simulink model "Simulation_Fahrmodell_v3"  (R2023b)
settings: Solver=ode14x  StartTime=0.0  StopTime=600  FixedStep=0.005  RelTol=1e-3
values from neighbouring files (symbols this model uses):
  bat = bat.computePack()    [DoE_main.m]    (also in DoE_main_sensitivity.m)
  cp = cp.computeP4Map(val_P4, 0, val_P4_DM, 0, 0)    [DoE_main.m]    (also in DoE_main_sensitivity.m = cp.computeP4Map(P4, E2, P4_DM, E3, E4))
  gb = gb.computeShiftMaps()    [DoE_main.m]    (also in DoE_main_sensitivity.m)
  P4 = cfgNum(cfg, 'P4', 0)    [DoE_main_sensitivity.m]    (also in PowertrainConfig.m = 0)
  P4_DM = cfgNum(cfg, 'P4_DM', 0)    [DoE_main_sensitivity.m]    (also in PowertrainConfig.m = 0)
  pt = pt.setupHybrid()    [DoE_main.m]    (also in DoE_main_sensitivity.m)
  veh = VehicleConfig()    [DoE_main.m]    (also in DoE_main_sensitivity.m)
undefined symbols (not defined in the file or in its folder): cp_Zelle_JpkgK, Ice_derfacLoadDecrease_MAP, Ice_derfacLoadIncrease_MAP, Ice_n_axis, Ice_relLoadMax_CUR_n, Ice_relLoadMax_CUR_val, Ice_rl_axis_norm, seconds, SKO_STREET_CHAL, SKO_WHEEL_TYP_CHAL, slip_pacejka, T_init_degC, Track, TT_sliced, use_turbo_model, v_Fzg_init_kmph
libraries: nesl_utility x15, fl_lib x9
(part 2 of 6)

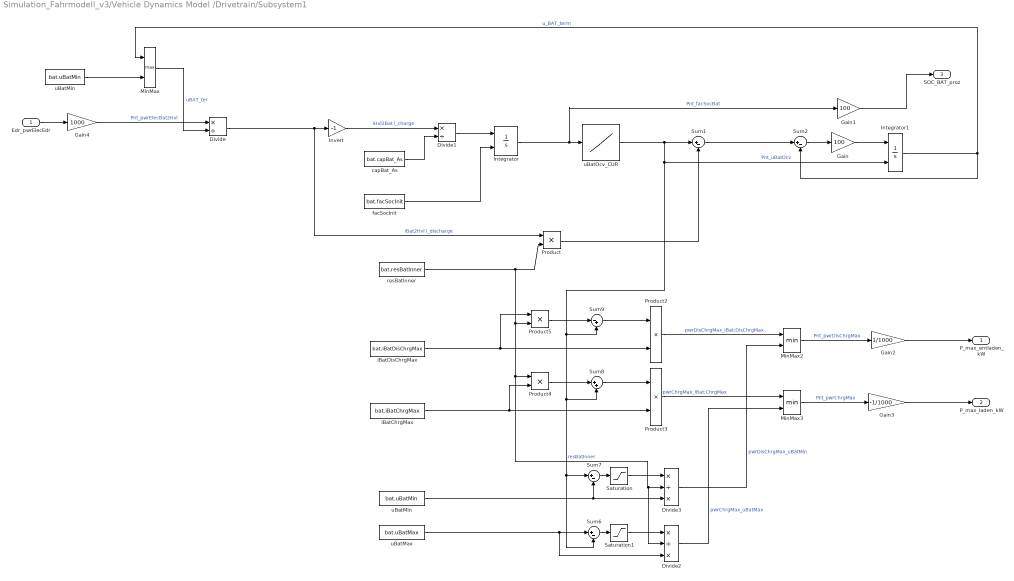
== system Simulation_Fahrmodell_v3/Vehicle Dynamics Model /Drivetrain/Subsystem1 ==
  Edr_pwrElecEdr : Inport
  Divide : Product  Inputs=*/
  Divide1 : Product  Inputs=*/
  Divide2 : Product  Inputs=*/*
  Divide3 : Product  Inputs=*/*
  Gain : Gain  Gain=100
  Gain1 : Gain  Gain=100
  Gain2 : Gain  Gain=1/1000
  Gain3 : Gain  Gain=-1/1000
  Gain4 : Gain  Gain=1000
  Integrator : Integrator  InitialConditionSource=external  InitialCondition=0.8  LimitOutput=on  UpperSaturationLimit=1  LowerSaturationLimit=0
  Integrator1 : Integrator  InitialConditionSource=external  InitialCondition=0.8
  Invert : Gain  Gain=-1
  MinMax : MinMax  Function=max  Inputs=2
  MinMax2 : MinMax  Inputs=2
  MinMax3 : MinMax  Inputs=2
  Product : Product  RndMeth=Zero
  Product{2..5} (4 alike) : Product
  Saturation : Saturate  UpperLimit=1000  LowerLimit=0
  Saturation1 : Saturate  UpperLimit=1000  LowerLimit=0
  Sum{1..2,6..7} (4 alike) : Sum  Inputs=|+-
  Sum8 : Sum  Inputs=|++
  Sum9 : Sum  Inputs=|-+
  capBat_As : Constant  Value=bat.capBat_As
  facSocInit : Constant  Value=bat.facSocInit
  iBatChrgMax : Constant  Value=bat.iBatChrgMax
  iBatDisChrgMax : Constant  Value=bat.iBatDisChrgMax
  resBatInner : Constant  Value=bat.resBatInner
  uBatMax : Constant  Value=bat.uBatMax
  uBatMin : Constant  Value=bat.uBatMin
  "uBatMin " : Constant  Value=bat.uBatMin
  uBatOcv_CUR : Lookup_n-D  NumberOfTableDimensions=1  BreakpointsForDimension1=bat.Soc_Axis  Table=bat.uBatOcv_Table  InternalRulePriority=Speed  RndMeth=Simplest
  P_max_entladen_kW : Outport  VectorParamsAs1DForOutWhenUnconnected=off
  P_max_laden_kW : Outport  Port=2  VectorParamsAs1DForOutWhenUnconnected=off
  SOC_BAT_proz : Outport  Port=3  VectorParamsAs1DForOutWhenUnconnected=off
  wires:
  Edr_pwrElecEdr/1 -> Gain4/1
  Gain4/1 -> Divide/1  "Pnt_pwrElecBat2Hvl"
  MinMax/1 -> Divide/2  "uBAT_ter"
  Divide/1 -> Product/1, Invert/1  "iBat2Hvl i_discharge"
  Invert/1 -> Divide1/1  "iHvl2Bat i_charge"
  capBat_As/1 -> Divide1/2
  facSocInit/1 -> Integrator/2
  Divide1/1 -> Integrator/1
  Integrator/1 -> Gain1/1, uBatOcv_CUR/1  "Pnt_facSocBat"
  uBatOcv_CUR/1 -> Sum9/2, Sum8/2, Sum7/1, Sum6/2, Integrator1/2, Sum1/1  "Pnt_uBatOcv"
  resBatInner/1 -> Product/2, Product5/2, Divide2/2, Divide3/2, Product4/1  "resBatInner"
  Product/1 -> Sum1/2
  iBatChrgMax/1 -> Product3/2, Product4/2
  iBatDisChrgMax/1 -> Product2/2, Product5/1
  Product5/1 -> Sum9/1
  Product4/1 -> Sum8/1
  Sum9/1 -> Product2/1
  Sum8/1 -> Product3/1
  Product2/1 -> MinMax2/1  "pwrDisChrgMax_iBat;DisChrgMax"
  Product3/1 -> MinMax3/1  "pwrChrgMax_iBat;ChrgMax"
  Saturation/1 -> Divide3/1
  Sum6/1 -> Saturation1/1
  uBatMax/1 -> Sum6/1, Divide2/3
  Saturation1/1 -> Divide2/1
  Sum7/1 -> Saturation/1
  "uBatMin "/1 -> Sum7/2, Divide3/3
  Divide3/1 -> MinMax2/2  "pwrDisChrgMax_uBatMin"
  Divide2/1 -> MinMax3/2  "pwrChrgMax_uBatMax"
  MinMax2/1 -> Gain2/1  "Pnt_pwrDisChrgMax"
  MinMax3/1 -> Gain3/1  "Pnt_pwrChrgMax"
  uBatMin/1 -> MinMax/2
  Integrator1/1 -> MinMax/1, Sum2/2  "u_BAT_term"
  Sum2/1 -> Gain/1
  Gain/1 -> Integrator1/1
  Sum1/1 -> Sum2/1
  Gain1/1 -> SOC_BAT_proz/1
  Gain2/1 -> P_max_entladen_kW/1
  Gain3/1 -> P_max_laden_kW/1

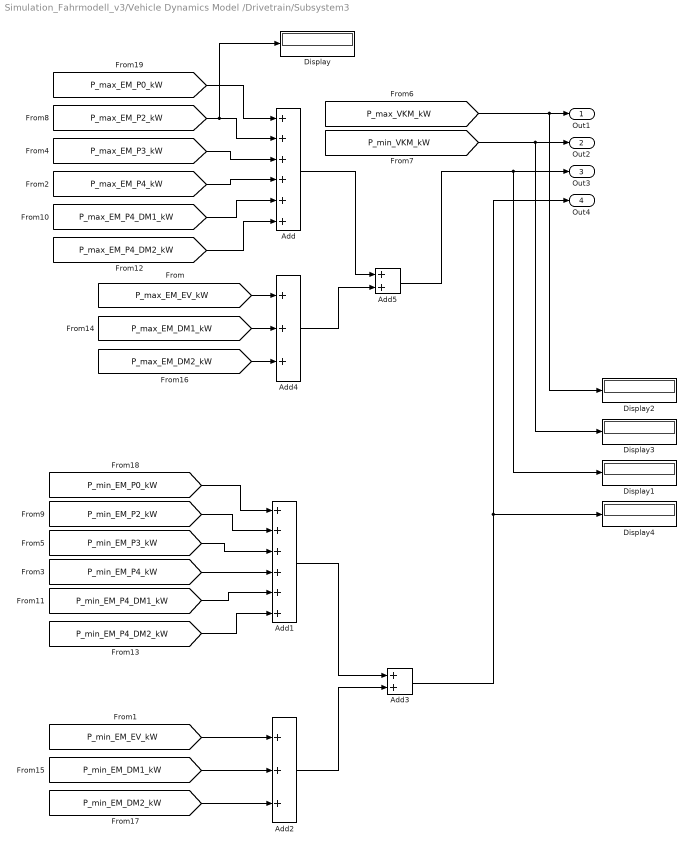
== system Simulation_Fahrmodell_v3/Vehicle Dynamics Model /Drivetrain/Subsystem3 ==
  Add : Sum  Inputs=++++++
  Add1 : Sum  Inputs=++++++
  Add2 : Sum  Inputs=+++
  Add3 : Sum
  Add4 : Sum  Inputs=+++
  Add5 : Sum
  Display{,1..4} (5 alike) : Display
  Out1 : Outport
  Out2 : Outport  Port=2
  Out3 : Outport  Port=3
  Out4 : Outport  Port=4
  wires:
  Add3/1 -> Out4/1, Display4/1
  Add1/1 -> Add3/1
  [P_min_EM_DM2_kW] -> Add2/3
  [P_min_EM_DM1_kW] -> Add2/2
  Add/1 -> Add5/1
  [P_max_EM_P4_DM1_kW] -> Add/5
  [P_max_EM_P3_kW] -> Add/3
  [P_max_EM_P0_kW] -> Add/1
  [P_max_EM_P2_kW] -> Add/2, Display/1
  [P_min_EM_EV_kW] -> Add2/1
  [P_min_EM_P4_DM2_kW] -> Add1/6
  [P_min_EM_P3_kW] -> Add1/3
  [P_max_EM_P4_kW] -> Add/4
  [P_max_EM_P4_DM2_kW] -> Add/6
  [P_min_EM_P0_kW] -> Add1/1
  Add2/1 -> Add3/2
  [P_min_VKM_kW] -> Out2/1, Display3/1
  [P_max_VKM_kW] -> Out1/1, Display2/1
  [P_min_EM_P4_DM1_kW] -> Add1/5
  [P_min_EM_P2_kW] -> Add1/2
  [P_min_EM_P4_kW] -> Add1/4
  [P_max_EM_DM1_kW] -> Add4/2
  [P_max_EM_EV_kW] -> Add4/1
  [P_max_EM_DM2_kW] -> Add4/3
  Add4/1 -> Add5/2
  Add5/1 -> Display1/1, Out3/1

== system Simulation_Fahrmodell_v3/Vehicle Dynamics Model /Drivetrain/Umrechung BAT -> EM 1 ==
  P_BAT_kW : Inport
  Add : Sum
  Constant6 : Constant  Value=0
  Gain4 : Gain  Gain=0.95
  Gain5 : Gain  Gain=0.95
  Gain6 : Gain  Gain=1/0.95
  Gain7 : Gain  Gain=1/0.95
  Max : MinMax  Function=max  Inputs=2
  Min4 : MinMax  Inputs=2
  P_EM_kW : Outport
  wires:
  Max/1 -> Gain4/1
  Constant6/1 -> Max/2, Min4/2
  P_BAT_kW/1 -> Max/1, Min4/1
  Gain5/1 -> Add/2
  Min4/1 -> Gain6/1
  Gain7/1 -> Add/1
  Add/1 -> P_EM_kW/1
  Gain6/1 -> Gain7/1
  Gain4/1 -> Gain5/1

== system Simulation_Fahrmodell_v3/Vehicle Dynamics Model /Drivetrain/Umrechung BAT -> EM 2 ==
  P_BAT_kW : Inport
  Add : Sum
  Constant6 : Constant  Value=0
  Gain4 : Gain  Gain=0.95
  Gain5 : Gain  Gain=0.95
  Gain6 : Gain  Gain=1/0.95
  Gain7 : Gain  Gain=1/0.95
  Max : MinMax  Function=max  Inputs=2
  Min4 : MinMax  Inputs=2
  P_EM_kW : Outport
  wires:
  Max/1 -> Gain4/1
  Constant6/1 -> Max/2, Min4/2
  P_BAT_kW/1 -> Max/1, Min4/1
  Gain5/1 -> Add/2
  Min4/1 -> Gain6/1
  Gain7/1 -> Add/1
  Add/1 -> P_EM_kW/1
  Gain6/1 -> Gain7/1
  Gain4/1 -> Gain5/1

== system Simulation_Fahrmodell_v3/Vehicle Dynamics Model /Drivetrain/Unterscheidung Regler und Gaspedal ==
  Regelfaktor : Inport
  Abs : Abs  SaturateOnIntegerOverflow=off
  Constant : Constant  Value=0
  Max : MinMax  Function=max  Inputs=2
  Gaspedalposition : Outport
  Regler : Outport  Port=2
  wires:
  Constant/1 -> Max/1
  Regelfaktor/1 -> Abs/1, Max/2
  Max/1 -> Gaspedalposition/1
  Abs/1 -> Regler/1

== system Simulation_Fahrmodell_v3/Vehicle Dynamics Model /Drivetrain/Wirkungsgrad Antriebsstrang Radebene -> Motorebene ==
  F_N IN : Inport
  Constant1 : Constant  Value=0.92
  Fahren : Product  Inputs=*/
  Reku : Product
  Switch1 : Switch  Criteria=u2 > Threshold  SaturateOnIntegerOverflow=off  InputSameDT=off
  F_N OUT : Outport
  wires:
  Constant1/1 -> Fahren/2, Reku/2
  F_N IN/1 -> Switch1/2, Fahren/1, Reku/1
  Reku/1 -> Switch1/3
  Switch1/1 -> F_N OUT/1
  Fahren/1 -> Switch1/1

== system Simulation_Fahrmodell_v3/Vehicle Dynamics Model /Drivetrain/v_mps -> v_kmph1 ==
  v_ist_mps IN : Inport
  Gain2 : Gain  Gain=3.6
  v_ist_kmph : Outport
  v_ist_mps OUT : Outport  Port=2
  wires:
  v_ist_mps IN/1 -> Gain2/1, v_ist_mps OUT/1
  Gain2/1 -> v_ist_kmph/1  "V_ist (km/h)"

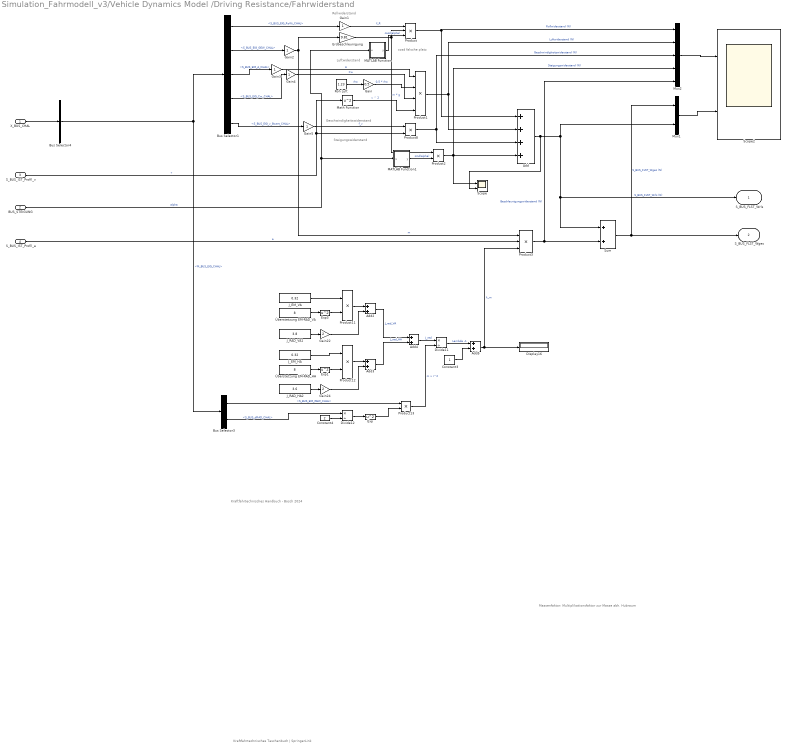
== system Simulation_Fahrmodell_v3/Vehicle Dynamics Model /Driving Resistance/Fahrwiderstand ==
  note: cosd falsche platz
  note: Kraftfahrtechnisches Taschenbuch | SpringerLink
  note: Kraftfahrtechnisches Handbuch - Bosch 2024
  note: Massenfaktor: Multiplikationsfaktor zur Masse abh. Hubraum
  note: Luftwiderstand
  note: Geschwindigkeitswiderstand
  note: Rollwiderstand
  note: Steigungswiderstand
  X_BUS_CHAL : Inport
  BUS_STEIGUNG : Inport  Port=2
  S_BUS_IST_Profil_v : Inport  Port=3
  S_BUS_IST_Profil_a : Inport  Port=4
  Add : Sum  Inputs=++++
  Add{2..5} (4 alike) : Sum
  Bus Selector1 : BusSelector  OutputSignals=S_BUS_EIG_RoWi_CHAL,S_BUS_EIG_GEW_CHAL,S_BUS_EIG_A_CHAL,S_BUS_EIG_Cw_CHAL,S_BUS_EIG_v_Bwert_CHAL
  Bus Selector3 : BusSelector  OutputSignals=S_BUS_EIG_GEW_CHAL,S_BUS_dRAD_CHAL
  Bus Selector4 : BusSelector  OutputSignals=M_BUS_EIG_CHAL
  Constant3 : Constant
  Constant4 : Constant  Value=2
  Display16 : Display
  Divide11 : Product  Inputs=*/
  Divide12 : Product  Inputs=*/
  Erdbeschleunigung : Gain  Gain=9.81
  Exp : Math  Operator=square
  Exp1 : Math  Operator=square
  Exp3 : Math  Operator=square
  Gain : Gain  Gain=0.5
  Gain{1..5} (5 alike) : Gain
  Gain22 : Gain  Gain=2
  Gain24 : Gain  Gain=2
  J_EM_HA : Constant  Value=0.32
  J_EM_VA : Constant  Value=0.32
  J_RAD_HA2 : Constant  Value=3.6
  J_RAD_VA1 : Constant  Value=3.8
  MATLAB Function : MATLAB Function  TreatAsAtomicUnit=on
  MATLAB Function1 : MATLAB Function  TreatAsAtomicUnit=on
  Math Function : Math  Operator=square
  Mux1 : Mux  Inputs=2
  Mux2 : Mux  Inputs=5
  Product : Product  Inputs=3
  Product1 : Product  Inputs=4
  Product{2,8,11..13} (5 alike) : Product
  Product3 : Product  Inputs=3
  Roh Luft : Constant  Value=1.23
  Scope : Scope  NumInputPorts=2
  Scope2 : Scope  NumInputPorts=2
  Sum : Sum
  Überstetzung EM-RAD_HA : Constant  Value=8
  Überstetzung EM-RAD_VA : Constant  Value=8
  S_BUS_FLST_Wrls : Outport
  S_BUS_FLST_Wges : Outport  Port=2
  wires:
  S_BUS_IST_Profil_a/1 -> Product3/2  "a"
  Bus Selector1/1 -> Gain1/1  "<S_BUS_EIG_RoWi_CHAL>"
  MATLAB Function/1(y) -> Product/3  "cosd(alpha)"
  Exp/1 -> Product13/2
  Math Function/1 -> Product1/4  "v ^ 2"
  MATLAB Function1/1(y) -> Product2/2  "sind(alpha)"
  BUS_STEIGUNG/1 -> MATLAB Function1/1(u), MATLAB Function/1(u)  "alpha"
  Bus Selector1/2 -> Gain2/1  "<S_BUS_EIG_GEW_CHAL>"
  Bus Selector1/3 -> Gain3/1  "<S_BUS_EIG_A_CHAL>"
  Product11/1 -> Add2/1
  Sum/1 -> S_BUS_FLST_Wges/1, Mux1/1  "S_BUS_FLST_Wges (N)"
  Erdbeschleunigung/1 -> Product2/1, Product/2  "m * g"
  Product13/1 -> Divide11/2  "m x r^2"
  Roh Luft/1 -> Gain/1  "rho"
  Product2/1 -> Add/4, Scope/1, Mux2/4  "Steigungswiderstand (N)"
  Product3/1 -> Sum/2, Mux2/5  "Beschleunigungswiderstand (N)"
  S_BUS_IST_Profil_v/1 -> Product8/2, Math Function/1  "v"
  Gain24/1 -> Add3/2
  Add/1 -> Scope/2, Mux1/2, Sum/1, S_BUS_FLST_Wrls/1  "S_BUS_FLST_Wrls (N)"
  Gain22/1 -> Add2/2
  J_EM_VA/1 -> Product11/1
  Mux2/1 -> Scope2/1
  Constant3/1 -> Add5/2
  Exp1/1 -> Product12/2
  Bus Selector1/5 -> Gain5/1  "<S_BUS_EIG_v_Bwert_CHAL>"
  Exp3/1 -> Product11/2
  Mux1/1 -> Scope2/2
  Bus Selector1/4 -> Gain4/1  "<S_BUS_EIG_Cw_CHAL>"
  Add4/1 -> Divide11/1  "J_red"
  Constant4/1 -> Divide12/2
  Product1/1 -> Mux2/2, Add/2  "Luftwiderstand (N)"
  Product/1 -> Add/1, Mux2/1  "Rollwiderstand (N)"
  Bus Selector3/2 -> Divide12/1  "<S_BUS_dRAD_CHAL>"
  Product12/1 -> Add3/1
  Gain/1 -> Product1/2  "0,5 * rho"
  Add2/1 -> Add4/1  "J_red_VA"
  Überstetzung EM-RAD_HA/1 -> Exp1/1
  J_RAD_VA1/1 -> Gain22/1
  Add5/1 -> Product3/3, Display16/1  "k_m"
  Add3/1 -> Add4/2  "J_rad_HA"
  J_EM_HA/1 -> Product12/1
  Divide12/1 -> Exp/1
  J_RAD_HA2/1 -> Gain24/1
  Überstetzung EM-RAD_VA/1 -> Exp3/1
  Product8/1 -> Add/3, Mux2/3  "Geschwindigkeitswiderstand (N)"
  Divide11/1 -> Add5/1  "Lambda -1"
  Bus Selector3/1 -> Product13/1  "<S_BUS_EIG_GEW_CHAL>"
  Bus Selector4/1 -> Bus Selector1/1, Bus Selector3/1  "<M_BUS_EIG_CHAL>"
  X_BUS_CHAL/1 -> Bus Selector4/1
  Gain1/1 -> Product/1  "f_R"
  Gain2/1 -> Product3/1, Erdbeschleunigung/1  "m"
  Gain3/1 -> Product1/1  "A"
  Gain4/1 -> Product1/3  "Cw"
  Gain5/1 -> Product8/1  "f_v"

== system Simulation_Fahrmodell_v3/Vehicle Dynamics Model /Driving Resistance/Subsystem ==
  X_BUS_CHAL : Inport
  BUS_STEIGUNG : Inport  Port=2
  M_m_Nm : Inport  Port=3
  Bus Selector2 : BusSelector  OutputSignals=M_BUS_EIG_CHAL.S_BUS_dRAD_CHAL
  Constant : Constant
  Delay1 : Delay  DelayLength=1
  Display{1..8} (8 alike) : Display
  Divide1 : Product  Inputs=*/
  Divide2 : Product  Inputs=*/
  Fahrwiderstand1 : Subsystem
  Integrator : Integrator
  Limit output 0..1 : Saturate  UpperLimit=1  LowerLimit=0
  Minus1 : Sum  Inputs=+-
  Minus2 : Sum  Inputs=+-
  Product{,1..3} (4 alike) : Product
  Scope2 : Scope  NumInputPorts=2
  Scope3 : Scope  NumInputPorts=2
  Test Konstante red. Massenträgheit : Constant  Value=65.92
  Tire Friction Model Pacejka Dry_tarmac : Lookup_n-D  NumberOfTableDimensions=1  BreakpointsForDimension1=slip_pacejka.Dry_tarmac.slip  Table=slip_pacejka.Dry_tarmac.y  UseLastTableValue=on  InternalRulePriority=Speed  RndMeth=Simplest
  "d -> r" : Gain  Gain=0.5
  g : Constant  Value=9.81
  m_kg : Constant  Value=2500
  wires:
  X_BUS_CHAL/1 -> Bus Selector2/1, Fahrwiderstand1/1(X_BUS_CHAL)
  M_m_Nm/1 -> Display2/1, Scope3/1, Minus2/1
  Fahrwiderstand1/1(v) -> Display8/1, Divide2/1  "v"
  Divide1/1 -> Integrator/1, Display1/1  "Winkelbeschleunigung Rad alpha_F"
  Divide2/1 -> Minus1/2
  Product3/1 -> Delay1/1  "Tire Force Disturbance"
  Minus1/1 -> Display4/1, Scope2/1, Limit output 0..1/1
  Test Konstante red. Massenträgheit/1 -> Divide1/2
  Tire Friction Model Pacejka Dry_tarmac/1 -> Display6/1, Product2/2  "Reibkoeffizient mu"
  "d -> r"/1 -> Display7/1, Product3/2, Product/2  "r"
  g/1 -> Product1/2
  Delay1/1 -> Scope3/2, Minus2/2, Display3/1
  m_kg/1 -> Product1/1
  Minus2/1 -> Divide1/1
  Limit output 0..1/1 -> Display5/1, Scope2/2, Tire Friction Model Pacejka Dry_tarmac/1  "Schlupf lambda"
  Bus Selector2/1 -> "d -> r"/1  "<S_BUS_dRAD_CHAL>"
  BUS_STEIGUNG/1 -> Fahrwiderstand1/2(BUS_STEIGUNG)
  Product2/1 -> Fahrwiderstand1/3(F_x_N), Product3/1  "F_x_N"
  Integrator/1 -> Product/1  "Winkelgeschwindigkeit Rad omega_F"
  Constant/1 -> Minus1/1
  Product1/1 -> Product2/1  "F_z_N"
  Product/1 -> Divide2/2  "omega_F * r"

== system Simulation_Fahrmodell_v3/Vehicle Properties/Fzg.-Eigenschaften/Eingabe i_GET und n_max_Upmin Andere Angaben ==
  Bus Creator : BusCreator  Inputs=8
  Bus Creator1 : BusCreator  Inputs=2
  Bus Creator2 : BusCreator  Inputs=8
  i_G1 : Constant  Value=i_G1
  i_G2 : Constant  Value=i_G2
  i_G3 : Constant  Value=i_G3
  i_G4 : Constant  Value=i_G4
  i_G5 : Constant  Value=i_G5
  i_G6 : Constant  Value=i_G6
  i_G7 : Constant  Value=i_G7
  i_G8 : Constant  Value=i_G8
  n_max_Upmin G1 : Constant  Value=n_max_Upmin_G1
  n_max_Upmin G2 : Constant  Value=n_max_Upmin_G2
  n_max_Upmin G3 : Constant  Value=n_max_Upmin_G3
  n_max_Upmin G4 : Constant  Value=n_max_Upmin_G4
  n_max_Upmin G5 : Constant  Value=n_max_Upmin_G5
  n_max_Upmin G6 : Constant  Value=n_max_Upmin_G6
  n_max_Upmin G7 HARTE GRENZE : Constant  Value=n_max_Upmin_G7
  n_max_Upmin G8 : Constant  Value=n_max_Upmin_G8
  BUS OUT : Outport
  wires:
  i_G1/1 -> Bus Creator/1  "G1"
  i_G2/1 -> Bus Creator/2  "G2"
  i_G3/1 -> Bus Creator/3  "G3"
  i_G4/1 -> Bus Creator/4  "G4"
  i_G5/1 -> Bus Creator/5  "G5"
  i_G6/1 -> Bus Creator/6  "G6"
  i_G7/1 -> Bus Creator/7  "G7"
  i_G8/1 -> Bus Creator/8  "G8"
  n_max_Upmin G1/1 -> Bus Creator2/1  "G1"
  n_max_Upmin G2/1 -> Bus Creator2/2  "G2"
  n_max_Upmin G6/1 -> Bus Creator2/6  "G6"
  n_max_Upmin G4/1 -> Bus Creator2/4  "G4"
  n_max_Upmin G3/1 -> Bus Creator2/3  "G3"
  n_max_Upmin G7 HARTE GRENZE/1 -> Bus Creator2/7  "G7"
  n_max_Upmin G5/1 -> Bus Creator2/5  "G5"
  n_max_Upmin G8/1 -> Bus Creator2/8  "G8"
  Bus Creator/1 -> Bus Creator1/1  "i_GET"
  Bus Creator2/1 -> Bus Creator1/2  "n_max_Upmin"
  Bus Creator1/1 -> BUS OUT/1

== system Simulation_Fahrmodell_v3/Vehicle Properties/Fzg.-Eigenschaften/Eingabe i_GET und n_max_Upmin Audi RS3 8YA PA ==
  Bus Creator : BusCreator  Inputs=8
  Bus Creator1 : BusCreator  Inputs=2
  Bus Creator2 : BusCreator  Inputs=8
  i_G1 : Constant  Value=i_G1
  i_G2 : Constant  Value=i_G2
  i_G3 : Constant  Value=i_G3
  i_G4 : Constant  Value=i_G4
  i_G5 : Constant  Value=i_G5
  i_G6 : Constant  Value=i_G6
  i_G7 : Constant  Value=i_G7
  i_G8 : Constant  Value=i_G8
  n_max_Upmin G1 : Constant  Value=n_max_Upmin_G1
  n_max_Upmin G2 : Constant  Value=n_max_Upmin_G2
  n_max_Upmin G3 : Constant  Value=n_max_Upmin_G3
  n_max_Upmin G4 : Constant  Value=n_max_Upmin_G4
  n_max_Upmin G5 : Constant  Value=n_max_Upmin_G5
  n_max_Upmin G6 : Constant  Value=n_max_Upmin_G6
  n_max_Upmin G7 HARTE GRENZE : Constant  Value=n_max_Upmin_G7
  n_max_Upmin G8 : Constant  Value=n_max_Upmin_G8
  BUS OUT : Outport
  wires:
  i_G1/1 -> Bus Creator/1  "G1"
  i_G2/1 -> Bus Creator/2  "G2"
  i_G3/1 -> Bus Creator/3  "G3"
  i_G4/1 -> Bus Creator/4  "G4"
  i_G5/1 -> Bus Creator/5  "G5"
  i_G6/1 -> Bus Creator/6  "G6"
  i_G7/1 -> Bus Creator/7  "G7"
  i_G8/1 -> Bus Creator/8  "G8"
  n_max_Upmin G1/1 -> Bus Creator2/1  "G1"
  n_max_Upmin G2/1 -> Bus Creator2/2  "G2"
  n_max_Upmin G6/1 -> Bus Creator2/6  "G6"
  n_max_Upmin G4/1 -> Bus Creator2/4  "G4"
  n_max_Upmin G3/1 -> Bus Creator2/3  "G3"
  n_max_Upmin G7 HARTE GRENZE/1 -> Bus Creator2/7  "G7"
  n_max_Upmin G5/1 -> Bus Creator2/5  "G5"
  n_max_Upmin G8/1 -> Bus Creator2/8  "G8"
  Bus Creator/1 -> Bus Creator1/1  "i_GET"
  Bus Creator2/1 -> Bus Creator1/2  "n_max_Upmin"
  Bus Creator1/1 -> BUS OUT/1

== system Simulation_Fahrmodell_v3/Vehicle Properties/Fzg.-Eigenschaften/Eingabe i_GET und n_max_Upmin Spreizung 7,0 ==
  Bus Creator : BusCreator  Inputs=8
  Bus Creator1 : BusCreator  Inputs=2
  Bus Creator2 : BusCreator  Inputs=8
  i_G1 : Constant  Value=i_G1
  i_G2 : Constant  Value=i_G2
  i_G3 : Constant  Value=i_G3
  i_G4 : Constant  Value=i_G4
  i_G5 : Constant  Value=i_G5
  i_G6 : Constant  Value=i_G6
  i_G7 : Constant  Value=i_G7
  i_G8 : Constant  Value=i_G8
  n_max_Upmin G1 : Constant  Value=n_max_Upmin_G1
  n_max_Upmin G2 : Constant  Value=n_max_Upmin_G2
  n_max_Upmin G3 : Constant  Value=n_max_Upmin_G3
  n_max_Upmin G4 : Constant  Value=n_max_Upmin_G4
  n_max_Upmin G5 : Constant  Value=n_max_Upmin_G5
  n_max_Upmin G6 : Constant  Value=n_max_Upmin_G6
  n_max_Upmin G7 HARTE GRENZE : Constant  Value=n_max_Upmin_G7
  n_max_Upmin G8 : Constant  Value=n_max_Upmin_G8
  BUS OUT : Outport
  wires:
  i_G1/1 -> Bus Creator/1  "G1"
  i_G2/1 -> Bus Creator/2  "G2"
  i_G3/1 -> Bus Creator/3  "G3"
  i_G4/1 -> Bus Creator/4  "G4"
  i_G5/1 -> Bus Creator/5  "G5"
  i_G6/1 -> Bus Creator/6  "G6"
  i_G7/1 -> Bus Creator/7  "G7"
  i_G8/1 -> Bus Creator/8  "G8"
  n_max_Upmin G1/1 -> Bus Creator2/1  "G1"
  n_max_Upmin G2/1 -> Bus Creator2/2  "G2"
  n_max_Upmin G6/1 -> Bus Creator2/6  "G6"
  n_max_Upmin G4/1 -> Bus Creator2/4  "G4"
  n_max_Upmin G3/1 -> Bus Creator2/3  "G3"
  n_max_Upmin G7 HARTE GRENZE/1 -> Bus Creator2/7  "G7"
  n_max_Upmin G5/1 -> Bus Creator2/5  "G5"
  n_max_Upmin G8/1 -> Bus Creator2/8  "G8"
  Bus Creator/1 -> Bus Creator1/1  "i_GET"
  Bus Creator2/1 -> Bus Creator1/2  "n_max_Upmin"
  Bus Creator1/1 -> BUS OUT/1

== system Simulation_Fahrmodell_v3/Vehicle Properties/Fzg.-Eigenschaften/Eingabe i_GET und n_max_Upmin Spreizung 7,8 ==
  Bus Creator : BusCreator  Inputs=8
  Bus Creator1 : BusCreator  Inputs=2
  Bus Creator2 : BusCreator  Inputs=8
  i_G1 : Constant  Value=i_G1
  i_G2 : Constant  Value=i_G2
  i_G3 : Constant  Value=i_G3
  i_G4 : Constant  Value=i_G4
  i_G5 : Constant  Value=i_G5
  i_G6 : Constant  Value=i_G6
  i_G7 : Constant  Value=i_G7
  i_G8 : Constant  Value=i_G8
  n_max_Upmin G1 : Constant  Value=n_max_Upmin_G1
  n_max_Upmin G2 : Constant  Value=n_max_Upmin_G2
  n_max_Upmin G3 : Constant  Value=n_max_Upmin_G3
  n_max_Upmin G4 : Constant  Value=n_max_Upmin_G4
  n_max_Upmin G5 : Constant  Value=n_max_Upmin_G5
  n_max_Upmin G6 : Constant  Value=n_max_Upmin_G6
  n_max_Upmin G7 HARTE GRENZE : Constant  Value=n_max_Upmin_G7
  n_max_Upmin G8 : Constant  Value=n_max_Upmin_G8
  BUS OUT : Outport
  wires:
  i_G1/1 -> Bus Creator/1  "G1"
  i_G2/1 -> Bus Creator/2  "G2"
  i_G3/1 -> Bus Creator/3  "G3"
  i_G4/1 -> Bus Creator/4  "G4"
  i_G5/1 -> Bus Creator/5  "G5"
  i_G6/1 -> Bus Creator/6  "G6"
  i_G7/1 -> Bus Creator/7  "G7"
  i_G8/1 -> Bus Creator/8  "G8"
  n_max_Upmin G1/1 -> Bus Creator2/1  "G1"
  n_max_Upmin G2/1 -> Bus Creator2/2  "G2"
  n_max_Upmin G6/1 -> Bus Creator2/6  "G6"
  n_max_Upmin G4/1 -> Bus Creator2/4  "G4"
  n_max_Upmin G3/1 -> Bus Creator2/3  "G3"
  n_max_Upmin G7 HARTE GRENZE/1 -> Bus Creator2/7  "G7"
  n_max_Upmin G5/1 -> Bus Creator2/5  "G5"
  n_max_Upmin G8/1 -> Bus Creator2/8  "G8"
  Bus Creator/1 -> Bus Creator1/1  "i_GET"
  Bus Creator2/1 -> Bus Creator1/2  "n_max_Upmin"
  Bus Creator1/1 -> BUS OUT/1

== system Simulation_Fahrmodell_v3/Environment/Nürburgring (M. Siesmann)/Vehicle Dynamics: Desired Speed (Kamm Circle)/Subsystem ==
  Clock2 : Clock
  Delay1 : Delay  DelayLength=1
  Minus1 : Sum  Inputs=+-
  delta_t_s : Outport
  wires:
  Delay1/1 -> Minus1/2
  Clock2/1 -> Delay1/1, Minus1/1
  Minus1/1 -> delta_t_s/1

== system Simulation_Fahrmodell_v3/Vehicle Dynamics Model /Drivetrain/Axle Load and Torque Distribution /Axle Torque Channel Router  ==
  Tq_Primary_axle : Inport
  Tq_Secondary_axle : Inport  Port=2
  Constant : Constant  Value=veh.HM_VA
  Constant1 : Constant  Value=0
  Constant3 : Constant  Value=pt.P4
  Constant4 : Constant  Value=pt.P4_DM
  OR1 : Logic  Operator=OR  IconShape=distinctive  AllPortsSameDT=off  OutDataTypeStr=boolean
  Switch{,1..4} (5 alike) : Switch  Criteria=u2 > Threshold  SaturateOnIntegerOverflow=off  InputSameDT=off
  Tq_FrontAxle : Outport
  Tq_RearAxle : Outport  Port=2
  wires:
  Tq_Primary_axle/1 -> Switch3/3, Switch1/3, Switch2/3, Switch/1
  Switch/1 -> Switch3/1
  Tq_Secondary_axle/1 -> Switch1/1, Switch/3
  Constant/1 -> Switch/2, Switch1/2
  Switch1/1 -> Switch2/1
  Switch2/1 -> Tq_RearAxle/1
  Switch4/1 -> Switch3/2, Switch2/2
  Switch3/1 -> Tq_FrontAxle/1
  Constant1/1 -> Switch4/1
  [P4_Deactivate] -> Switch4/2
  OR1/1 -> Switch4/3
  Constant3/1 -> OR1/1
  Constant4/1 -> OR1/2

== system Simulation_Fahrmodell_v3/Vehicle Dynamics Model /Drivetrain/Axle Load and Torque Distribution /Berechnung Max. Radlast VA//HA aufgrund Reifen//Fahrbahn ==
  F_Haftgrenze [N] : Inport
  Raddurchmesser [m] : Inport  Port=2
  axle_load_FrontAxle [%] : Inport  Port=3
  axle_load_RearAxle [%] : Inport  Port=4
  Gain : Gain  Gain=0.01
  Gain1 : Gain  Gain=0.01
  Product : Product
  Product1 : Product
  Radlast HA : Product
  Radlast VA : Product
  Scope : Scope  NumInputPorts=2
  Scope1 : Scope  NumInputPorts=2
  "d -> r" : Gain  Gain=0.5
  Max. Radlast VA [Nm] aufgrund Reifen/Fahrbahn : Outport
  Max. Radlast HA [Nm] aufgrund Reifen/Fahrbahn : Outport  Port=2
  wires:
  axle_load_FrontAxle [%]/1 -> Gain/1
  axle_load_RearAxle [%]/1 -> Gain1/1
  Radlast HA/1 -> Product1/1
  Radlast VA/1 -> Product/1
  F_Haftgrenze [N]/1 -> Scope1/1, Radlast VA/1, Radlast HA/1
  "d -> r"/1 -> Product1/2, Product/2
  Raddurchmesser [m]/1 -> "d -> r"/1
  Product/1 -> Scope/1, Max. Radlast VA [Nm] aufgrund Reifen/Fahrbahn/1
  Product1/1 -> Max. Radlast HA [Nm] aufgrund Reifen/Fahrbahn/1, Scope/2
  Gain/1 -> Radlast VA/2
  Gain1/1 -> Radlast HA/2

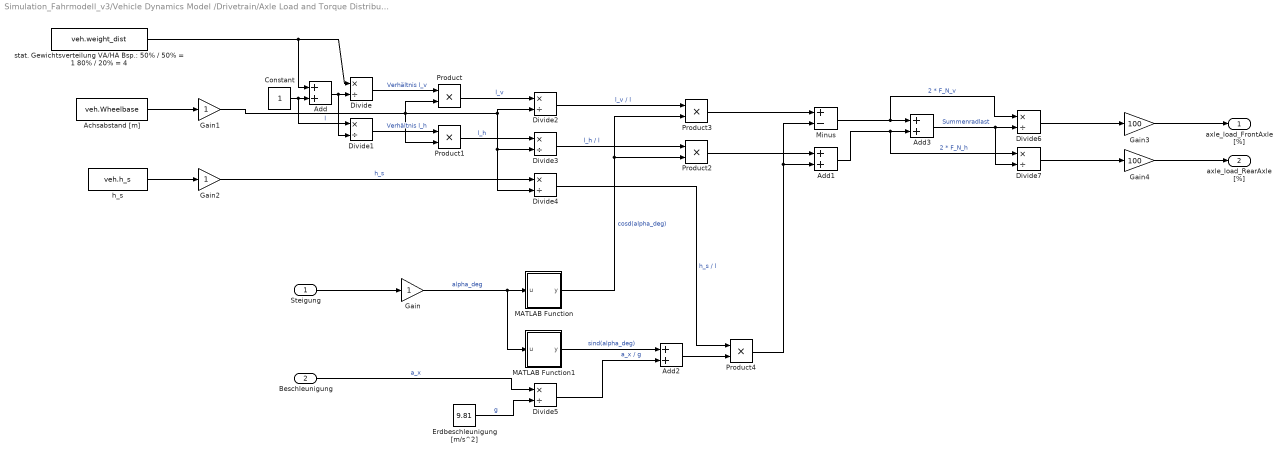
== system Simulation_Fahrmodell_v3/Vehicle Dynamics Model /Drivetrain/Axle Load and Torque Distribution /Berechnung Achslastverteilung abh. Fahrzeugeigenschaften (Haken Abs. 11) ==
  Steigung : Inport
  Beschleunigung : Inport  Port=2
  Achsabstand [m] : Constant  Value=veh.Wheelbase
  Add{,1..3} (4 alike) : Sum
  Constant : Constant
  Divide{,1..7} (8 alike) : Product  Inputs=*/
  Erdbeschleunigung [m/s^2] : Constant  Value=9.81
  Gain : Gain
  Gain1 : Gain
  Gain2 : Gain
  Gain3 : Gain  Gain=100
  Gain4 : Gain  Gain=100
  MATLAB Function : MATLAB Function  TreatAsAtomicUnit=on
  MATLAB Function1 : MATLAB Function  TreatAsAtomicUnit=on
  Minus : Sum  Inputs=+-
  Product{,1..4} (5 alike) : Product
  h_s : Constant  Value=veh.h_s
  stat. Gewichtsverteilung VA/HA Bsp.: 50% / 50% = 1 80% / 20% = 4 : Constant  Value=veh.weight_dist
  axle_load_FrontAxle [%] : Outport
  axle_load_RearAxle [%] : Outport  Port=2
  wires:
  Gain/1 -> MATLAB Function1/1(u), MATLAB Function/1(u)  "alpha_deg"
  Achsabstand [m]/1 -> Gain1/1
  Gain1/1 -> Divide4/2, Divide3/2, Divide2/2, Product1/2, Product/2  "l"
  Constant/1 -> Divide1/1, Add/2
  Add/1 -> Divide1/2, Divide/2
  stat. Gewichtsverteilung VA/HA Bsp.: 50% / 50% = 1 80% / 20% = 4/1 -> Divide/1, Add/1
  Divide/1 -> Product/1  "Verhältnis l_v"
  Divide1/1 -> Product1/1  "Verhältnis l_h"
  Product/1 -> Divide2/1  "l_v"
  Product1/1 -> Divide3/1  "l_h"
  MATLAB Function/1(y) -> Product3/2, Product2/2  "cosd(alpha_deg)"
  MATLAB Function1/1(y) -> Add2/1  "sind(alpha_deg)"
  Divide2/1 -> Product3/1  "l_v / l"
  Divide3/1 -> Product2/1  "l_h / l"
  h_s/1 -> Gain2/1
  Gain2/1 -> Divide4/1  "h_s"
  Divide4/1 -> Product4/1  "h_s / l"
  Beschleunigung/1 -> Divide5/1  "a_x"
  Erdbeschleunigung [m/s^2]/1 -> Divide5/2  "g"
  Divide5/1 -> Add2/2  "a_x / g"
  Product3/1 -> Minus/1
  Product2/1 -> Add1/1
  Add2/1 -> Product4/2
  Product4/1 -> Minus/2, Add1/2
  Minus/1 -> Divide6/1, Add3/1  "2 * F_N_v"
  Add1/1 -> Divide7/1, Add3/2  "2 * F_N_h"
  Divide6/1 -> Gain3/1
  Steigung/1 -> Gain/1
  Add3/1 -> Divide7/2, Divide6/2  "Summenradlast"
  Gain3/1 -> axle_load_FrontAxle [%]/1
  Divide7/1 -> Gain4/1
  Gain4/1 -> axle_load_RearAxle [%]/1

== system Simulation_Fahrmodell_v3/Vehicle Dynamics Model /Drivetrain/Axle Load and Torque Distribution /Drive Topology Axle Load Distributor  ==
  axle_load_FrontAxle [%] : Inport
  axle_load_RearAxle [%] : Inport  Port=2
  Tq_max_FrontAxle : Inport  Port=3
  Tq_max_RearAxle : Inport  Port=4
  Angetriebene Räder 1: Allrad 2: Hinterradantrieb 3: Vorderradantrieb : Constant  Commented=on  Value=3
  Constant : Constant  Value=0
  Constant1 : Constant  Value=0
  Constant2 : Constant  Value=pt.P4
  Constant3 : Constant  Value=veh.HM_VA
  Constant4 : Constant  Value=veh.AWD
  Constant5 : Constant  Value=pt.P4_DM
  Display : Display
  Display1 : Display
  Display2 : Display
  "Front Axle Load Calculator " : Subsystem
  MATLAB Function : MATLAB Function  TreatAsAtomicUnit=on
  Min2 : MinMax  Inputs=2
  Min3 : MinMax  Inputs=2
  Multiport Switch : MultiPortSwitch  SaturateOnIntegerOverflow=off  InputSameDT=off
  Multiport Switch1 : MultiPortSwitch  SaturateOnIntegerOverflow=off  InputSameDT=off
  OR1 : Logic  Operator=OR  IconShape=distinctive  AllPortsSameDT=off  OutDataTypeStr=boolean
  P4 AWD or AWD : Subsystem
  P4 AWD or AWD1 : Subsystem
  "Rear Axle Load Calculator " : Subsystem
  M_VA_Nm OUT : Outport
  M_HA_Nm OUT : Outport  Port=2
  wires:
  axle_load_FrontAxle [%]/1 -> "Rear Axle Load Calculator "/2(Achslast VA [%])
  Tq_max_RearAxle/1 -> "Rear Axle Load Calculator "/1(M_Nm), Min3/2, P4 AWD or AWD1/2(M_VA_Nm IN), Multiport Switch1/3
  "Rear Axle Load Calculator "/1(Radlast VA [Nm]) -> Min2/2
  Tq_max_FrontAxle/1 -> "Front Axle Load Calculator "/1(M_Nm), Multiport Switch/4, P4 AWD or AWD/1(M_VA_Nm IN), Min2/1
  axle_load_RearAxle [%]/1 -> "Front Axle Load Calculator "/2(Achslast HA [%])
  "Front Axle Load Calculator "/1(Radlast HA [Nm]) -> Min3/1
  Min2/1 -> Display/1, P4 AWD or AWD/2(In3)
  MATLAB Function/1(Driven_Wheels_Val) -> Multiport Switch1/1, Multiport Switch/1
  Multiport Switch/1 -> M_VA_Nm OUT/1
  Multiport Switch1/1 -> M_HA_Nm OUT/1
  Min3/1 -> P4 AWD or AWD1/3(In3), Display1/1
  Constant/1 -> Multiport Switch/3
  Constant1/1 -> Multiport Switch1/4
  Constant3/1 -> MATLAB Function/2(FWD)
  Constant4/1 -> MATLAB Function/1(AWD)
  Constant5/1 -> OR1/2
  Constant2/1 -> OR1/1
  OR1/1 -> P4 AWD or AWD1/1(In2), P4 AWD or AWD/3(In2), Display2/1, MATLAB Function/3(Check_P4)
  P4 AWD or AWD/1(Out1) -> Multiport Switch/2
  P4 AWD or AWD1/1(Out1) -> Multiport Switch1/2

== system Simulation_Fahrmodell_v3/Vehicle Dynamics Model /Drivetrain/Axle Load and Torque Distribution /Subsystem ==
  In1 : Inport
  In2 : Inport  Port=2
  "Tq_FrontAxle " : Inport  Port=3
  "Tq_RearAxle " : Inport  Port=4
  Gain{,1..3} (4 alike) : Gain  Gain=-1
  Max. Achslast HA [Nm] aufgrund Bauteilschutz : Constant  Value=8900
  Max. Achslast VA [Nm] aufgrund Bauteilschutz : Constant  Value=99999
  Min : MinMax  Inputs=3
  Min1 : MinMax  Inputs=3
  Min2 : MinMax  Function=max  Inputs=3
  Min3 : MinMax  Function=max  Inputs=3
  Tq_max_FrontAxle : Outport
  Tq_max_RearAxle : Outport  Port=2
  wires:
  Gain1/1 -> Min2/3
  Min/1 -> Min2/1
  In1/1 -> Min/2, Gain/1
  In2/1 -> Gain2/1, Min1/2
  Min1/1 -> Min3/1
  Max. Achslast HA [Nm] aufgrund Bauteilschutz/1 -> Gain3/1, Min1/3
  Gain3/1 -> Min3/3
  Max. Achslast VA [Nm] aufgrund Bauteilschutz/1 -> Gain1/1, Min/3
  Gain2/1 -> Min3/2
  Gain/1 -> Min2/2
  Min2/1 -> Tq_max_FrontAxle/1  "M_VA_Nm IN"
  "Tq_FrontAxle "/1 -> Min/1
  Min3/1 -> Tq_max_RearAxle/1  "M_HA_Nm IN"
  "Tq_RearAxle "/1 -> Min1/1

== system Simulation_Fahrmodell_v3/Vehicle Dynamics Model /Drivetrain/GETRIEBE auswahl VK, EV/Subsystem ==
  d_Rad_m : Inport
  Display4 : Display
  "d -> r" : Gain  Gain=0.5
  "m -> mm" : Gain  Gain=1000
  r_dyn_mm : Outport
  wires:
  d_Rad_m/1 -> "m -> mm"/1, Display4/1
  "d -> r"/1 -> r_dyn_mm/1
  "m -> mm"/1 -> "d -> r"/1

== system Simulation_Fahrmodell_v3/Vehicle Dynamics Model /Drivetrain/GETRIEBE auswahl VK, EV/Transmission Selector ==
  note: 1) Add Subsystem or Model blocks as valid variant choices.
      | 2) You cannot connect blocks at this level. At simulation, connectivity is automatically
      | determined, based on the active variant and port name matching.
  n_mot_Upmin : Inport
  i_AG : Inport  Port=2
  "Gaspedalposition [0, 1]" : Inport  Port=3
  " EV Single-Speed" : Subsystem  VariantControl=veh.EV == 1
  ICE Multi-Speed : Subsystem  VariantControl=veh.VM == 1 || veh.Hy ==1
  i_GES : Outport
  i_GES_delay : Outport  Port=2

== system Simulation_Fahrmodell_v3/Vehicle Dynamics Model /Drivetrain/GETRIEBE auswahl VK, EV/v_Fzg_kmph -> n_mot_Upmin ==
  i_GES : Inport
  r_dyn_mm : Inport  Port=2
  v_Fzg_kmph : Inport  Port=3
  Radschlupf : Inport  Port=4
  Constant : Constant  Value=2*pi*60/1000
  Divide : Product  Inputs=*/
  Product : Product
  Product1 : Product
  Product2 : Product
  "mm -> m" : Gain  Gain=0.001
  n_mot_Upmin : Outport
  wires:
  Product2/1 -> Product/1  "v_ist (km/h)"
  Radschlupf/1 -> Product2/1  "v_ist (km/h)"
  Divide/1 -> n_mot_Upmin/1
  Product1/1 -> Divide/2
  Constant/1 -> Product1/2
  Product/1 -> Divide/1
  i_GES/1 -> Product/2
  v_Fzg_kmph/1 -> Product2/2
  "mm -> m"/1 -> Product1/1
  r_dyn_mm/1 -> "mm -> m"/1

== system Simulation_Fahrmodell_v3/Vehicle Dynamics Model /Drivetrain/Operating Strategy 1.1/Axle Torque Split ==
  tq_wheel_des : Inport
  SOC : Inport  Port=2
  Add : Sum
  Constant1 : Constant  Value=pt.cfg_P4
  Constant2 : Constant  Value=veh.MainAxle_TorqueSplit_int
  Constant3 : Constant  Value=pt.cfg_P4_DM
  Constant4 : Constant  Value=gb.i_ges_P4
  Constant5 : Constant  Value=veh.EV
  Display : Display
  Display1 : Display
  Gain2 : Gain  Gain=0.01
  MATLAB Function1 : MATLAB Function  TreatAsAtomicUnit=on
  Min : MinMax  Inputs=2
  OR : Logic  Operator=OR  IconShape=distinctive  AllPortsSameDT=off  OutDataTypeStr=boolean
  Product : Product
  Product1 : Product
  Product4 : Product
  Saturation : Saturate  UpperLimit=10000  LowerLimit=0
  Subtract : Sum  Inputs=+-
  tq_wheel_Primary_axle_des : Outport
  tq_wheel_Secondary_axle_des : Outport  Port=2
  tag scope: P4_Deactivate=global
  wires:
  Product4/1 -> Min/2, Subtract/2  "tq_wheel_P4_max"
  Min/1 -> Display/1, tq_wheel_Secondary_axle_des/1  "tq_wheel_P4_des"
  Saturation/1 -> Add/2
  [tq_sh_P4_max] -> Product4/1
  Constant4/1 -> Product4/2
  Subtract/1 -> Saturation/1
  Add/1 -> tq_wheel_Primary_axle_des/1  "tq_wheel_ICEaxle_des"
  Product/1 -> Add/1  "tq_wheel_ICEaxle_des"
  Product1/1 -> Min/1, Subtract/1  "tq_wheel_P4axle_des"
  tq_wheel_des/1 -> Product1/2, Product/2  "tq_wheel_des"
  MATLAB Function1/2(Torque_ICE_Axle_percent) -> Product/1
  MATLAB Function1/3(Torque_P4_Axle_percent) -> Product1/1
  SOC/1 -> Gain2/1
  OR/1 -> MATLAB Function1/2(cfg_P4)
  Constant2/1 -> MATLAB Function1/4(MainAxle_TorqueSplit_int)
  Gain2/1 -> MATLAB Function1/1(SOC)
  Constant1/1 -> OR/1
  Constant3/1 -> OR/2
  Constant5/1 -> MATLAB Function1/3(EV)
  MATLAB Function1/1(P4_deactivate) -> [P4_Deactivate], Display1/1

== system Simulation_Fahrmodell_v3/Vehicle Dynamics Model /Drivetrain/Operating Strategy 1.1/EMs Priority (Ep) ==
  tq_wheel_Primary_axle_des : Inport
  i_ges : Inport  Port=2
  i_AG : Inport  Port=3
  SOC : Inport  Port=4
  Add1 : Sum  Inputs=+++
  Add2 : Sum  Inputs=+-
  MATLAB Function : MATLAB Function  TreatAsAtomicUnit=on  SystemSampleTime=0.01
  Min1 : MinMax  Inputs=2
  Product1 : Product
  Product2 : Product
  Product3 : Product
  SOC LIMIT : Subsystem  Commented=on
  Saturation : Saturate  UpperLimit=inf  LowerLimit=0
  tq_wheel_Elec_des_Ep : Outport
  tq_wheel_ICE_des_Ep : Outport  Port=2
  wires:
  tq_wheel_Primary_axle_des/1 -> Add2/1, Min1/2
  i_ges/1 -> Product2/1, Product1/1
  Add1/1 -> Min1/1, Add2/2
  [tq_sh_P2_max] -> Product2/2
  Product2/1 -> Add1/2  "tq_wheel_P2_max"
  Add2/1 -> Saturation/1
  Product3/1 -> Add1/3  "tq_wheel_P3_max"
  [tq_sh_P3_max] -> Product3/2
  Product1/1 -> Add1/1  "tq_wheel_P0_max"
  [tq_sh_P0_max] -> Product1/2
  i_AG/1 -> Product3/1
  Saturation/1 -> MATLAB Function/1(tq_ICE_in)  "tq_wheel_ICE_des_Ep"
  SOC/1 -> MATLAB Function/3(SOC)
  Min1/1 -> MATLAB Function/2(tq_Elec_in)  "tq_wheel_Elec_des_Ep"
  MATLAB Function/1(tq_ICE_out) -> tq_wheel_ICE_des_Ep/1
  MATLAB Function/2(tq_Elec_out) -> tq_wheel_Elec_des_Ep/1

== system Simulation_Fahrmodell_v3/Vehicle Dynamics Model /Drivetrain/Operating Strategy 1.1/ICE Priority (ICEp) ==
  tq_wheel_Primary_axle_des : Inport
  i_ges : Inport  Port=2
  Add : Sum  Inputs=+-
  Min : MinMax  Inputs=2
  Product : Product
  Saturation : Saturate  UpperLimit=inf  LowerLimit=0
  tq_wheel_Elec_des_ICEp : Outport
  tq_wheel_ICE_des_ICEp : Outport  Port=2
  wires:
  [tq_sh_ICE_max] -> Product/2
  tq_wheel_Primary_axle_des/1 -> Min/1, Add/1
  Min/1 -> tq_wheel_ICE_des_ICEp/1  "tq_wheel_ICE_des"
  Add/1 -> Saturation/1
  Saturation/1 -> tq_wheel_Elec_des_ICEp/1  "tq_wheel_Elec_des"
  Product/1 -> Min/2, Add/2  "tq_wheel_ICE_max"
  i_ges/1 -> Product/1

== system Simulation_Fahrmodell_v3/Vehicle Dynamics Model /Drivetrain/Operating Strategy 1.1/Priority Mode Output Combiner ==
  tq_wheel_Elec_des_ICEp : Inport
  tq_wheel_ICE_des_ICEp : Inport  Port=2
  tq_wheel_Elec_des_Ep : Inport  Port=3
  tq_wheel_ICE_des_Ep : Inport  Port=4
  Add : Sum
  Constant1 : Constant  Value=veh.VM
  Constant3 : Constant  Value=veh.Hybrid_ICE_priority
  Switch1 : Switch  Criteria=u2 > Threshold  SaturateOnIntegerOverflow=off  InputSameDT=off
  Switch2 : Switch  Criteria=u2 > Threshold  SaturateOnIntegerOverflow=off  InputSameDT=off
  Switch3 : Switch  Criteria=u2 > Threshold  SaturateOnIntegerOverflow=off  InputSameDT=off
  tq_wheel_ICE_des : Outport
  tq_wheel_Elec_des : Outport  Port=2
  wires:
  Add/1 -> Switch3/1
  Switch2/1 -> Switch3/3, Add/2
  Switch1/1 -> tq_wheel_Elec_des/1, Add/1
  Constant3/1 -> Switch1/2, Switch2/2
  tq_wheel_ICE_des_ICEp/1 -> Switch2/1
  tq_wheel_Elec_des_ICEp/1 -> Switch1/1
  tq_wheel_ICE_des_Ep/1 -> Switch2/3
  tq_wheel_Elec_des_Ep/1 -> Switch1/3
  Switch3/1 -> tq_wheel_ICE_des/1  "tq_wheel_ICE_des"
  Constant1/1 -> Switch3/2

== system Simulation_Fahrmodell_v3/Vehicle Dynamics Model /Drivetrain/Operating Strategy 1.1/Wheel-to-Shaft Converter and Demand Validators  ==
  i_ges : Inport
  i_AG : Inport  Port=2
  tq_wheel_ICE_des : Inport  Port=3
  tq_wheel_P0_des : Inport  Port=4
  tq_wheel_P2_des : Inport  Port=5
  tq_wheel_P3_des : Inport  Port=6
  tq_wheel_Primary_axle_des : Inport  Port=7
  tq_wheel_Secondary_axle_des : Inport  Port=8
  Bus Creator : BusCreator  Inputs=6
  Constant3 : Constant  Value=gb.i_ges_P4
  Constant4 : Constant  Value=gb.i_GET_EV
  Divide{,1..5} (6 alike) : Product  Inputs=*/
  EV Primary Axle Torque Path Selector : Subsystem
  Secondary Axle Torque Path Selector : Subsystem
  tq_sh_des : Outport
  wires:
  i_ges/1 -> Divide/2, Divide1/2, Divide3/2
  tq_wheel_ICE_des/1 -> Divide3/1
  tq_wheel_P3_des/1 -> Divide2/1
  tq_wheel_P0_des/1 -> Divide/1
  Constant3/1 -> Divide4/2
  i_AG/1 -> Divide2/2
  tq_wheel_P2_des/1 -> Divide1/1
  Divide1/1 -> Bus Creator/3  "tq_sh_P2_des"
  Divide3/1 -> Bus Creator/1  "tq_sh_ICE_des"
  Divide/1 -> Bus Creator/2  "tq_sh_P0_des"
  Divide2/1 -> Bus Creator/4  "tq_sh_P3_des"
  Divide4/1 -> Bus Creator/5  "tq_sh_P4_des"
  Divide5/1 -> Bus Creator/6  "tq_sh_EV_des"
  Bus Creator/1 -> tq_sh_des/1
  tq_wheel_Primary_axle_des/1 -> Secondary Axle Torque Path Selector/1(tq_wheel_Primary_axle_des), EV Primary Axle Torque Path Selector/1(tq_wheel_Primary_axle_des)
  Constant4/1 -> Divide5/2
  EV Primary Axle Torque Path Selector/1(tq_wheel_EV_des) -> Divide5/1
  tq_wheel_Secondary_axle_des/1 -> Secondary Axle Torque Path Selector/2(tq_wheel_Secondary_axle_des)
  Secondary Axle Torque Path Selector/1(tq_wheel_P4_des) -> Divide4/1

== system Simulation_Fahrmodell_v3/Vehicle Dynamics Model /Drivetrain/Primary and Secondary Axle Powertrain Selector/Primary Axle Powertrain Selector ==
  note: 1) Add Subsystem or Model blocks as valid variant choices.
      | 2) You cannot connect blocks at this level. At simulation, connectivity is automatically
      | determined, based on the active variant and port name matching.
  i_ges : Inport
  iAG : Inport  Port=2
  n_mot_Upmin : Inport  Port=3
  Regelfaktor : Inport  Port=4
  Torque_sh : Inport  Port=5
  Electric Drive : Subsystem  VariantControl=veh.EV == 1
  Hybrid Drive : Subsystem  VariantControl=veh.Hy == 1 || veh.VM == 1
  Tq_Primary_axle : Outport

== system Simulation_Fahrmodell_v3/Vehicle Dynamics Model /Drivetrain/Primary and Secondary Axle Powertrain Selector/Secondary Axle Powertrain Selector ==
  Regelfaktor1 : Inport
  n_mot_Upmin : Inport  Port=2
  iAG : Inport  Port=3
  i_ges : Inport  Port=4
  Torque_sh : Inport  Port=5
  Auswahl P4 : Switch  Commented=on  Criteria=u2 > Threshold  SaturateOnIntegerOverflow=off  InputSameDT=off
  "Auswahl P4, P4_Dual-Motor" : Subsystem  Variant=on
  Constant : Constant  Commented=on  Value=P4
  Constant1 : Constant  Commented=on  Value=0
  Constant2 : Constant  Commented=on  Value=P4_DM
  Constant3 : Constant  Commented=on  Value=0
  From : From  Commented=on  GotoTag=P4_Deactivate  TagVisibility=global
  OR : Logic  Commented=on  Operator=OR  IconShape=distinctive  AllPortsSameDT=off  OutDataTypeStr=boolean
  Switch : Switch  Commented=on  Criteria=u2 > Threshold  SaturateOnIntegerOverflow=off  InputSameDT=off
  Tq_Secondary_axle : Outport
  wires:
  Regelfaktor1/1 -> "Auswahl P4, P4_Dual-Motor"/2(Regelfaktor1)  "Regelfaktor1"
  iAG/1 -> "Auswahl P4, P4_Dual-Motor"/3(iAG)  "iAG"
  "Auswahl P4, P4_Dual-Motor"/1(M_Nm GET P4) -> Tq_Secondary_axle/1  "Gesamtmoment motorseitig"
  Constant1/1 -> Auswahl P4/3
  OR/1 -> Auswahl P4/2
  i_ges/1 -> "Auswahl P4, P4_Dual-Motor"/4(i_ges)
  Constant/1 -> OR/1
  Constant2/1 -> OR/2
  Torque_sh/1 -> "Auswahl P4, P4_Dual-Motor"/5(Torque_sh)
  Constant3/1 -> Switch/1
  n_mot_Upmin/1 -> "Auswahl P4, P4_Dual-Motor"/1(n_mot_Upmin)
  From/1 -> Switch/2

== system Simulation_Fahrmodell_v3/Vehicle Dynamics Model /Drivetrain/Reifenmodell1/Berechnung max. Radlast [N] ==
  mü eff (s,FB;RF)1 : Inport
  X_BUS_CHAL : Inport  Port=2
  Bus Selector1 : BusSelector  OutputSignals=M_BUS_EIG_CHAL.S_BUS_EIG_GEW_CHAL
  Display5 : Display
  Product : Product  Inputs=3
  g (m/s^2) : Constant  Value=9.81
  F_Haftgrenze (N) : Outport
  wires:
  g (m/s^2)/1 -> Product/2  "g (m/s^2)"
  mü eff (s,FB;RF)1/1 -> Product/3
  X_BUS_CHAL/1 -> Bus Selector1/1
  Bus Selector1/1 -> Product/1, Display5/1  "<S_BUS_EIG_GEW_CHAL>"
  Product/1 -> F_Haftgrenze (N)/1  "F_Haftgrenze (N)"

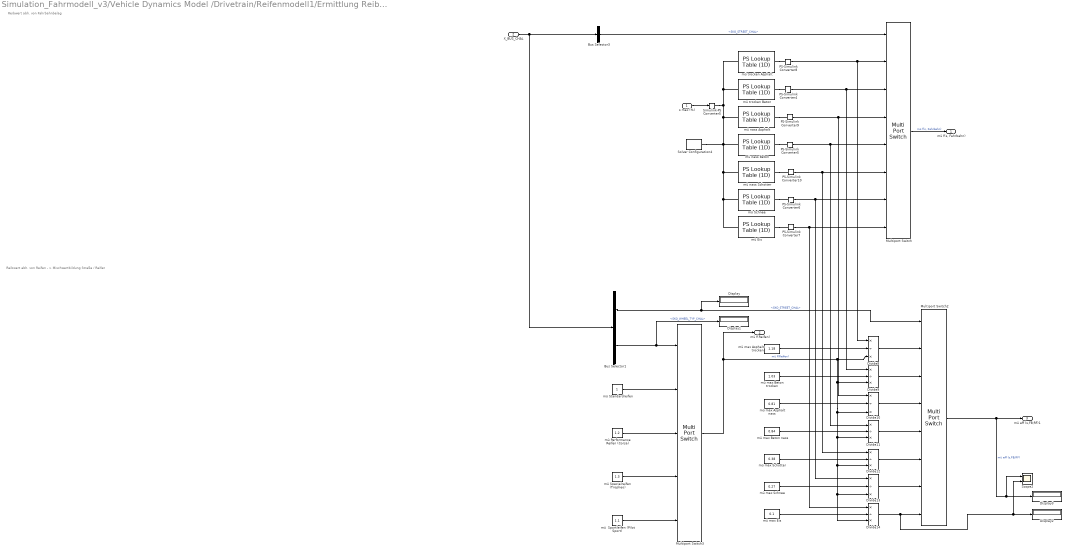
== system Simulation_Fahrmodell_v3/Vehicle Dynamics Model /Drivetrain/Reifenmodell1/Ermittlung Reibwert Abhängig von Fahrbahn und Reifen ==
  note: Reibwert abh. von Fahrbahnbelag
  note: Reibwert abh. von Reifen - > Mischwertbildung Straße / Reifen
  s max (%) : Inport
  X_BUS_CHAL : Inport  Port=2
  Bus Selector1 : BusSelector  OutputSignals=M_BUS_SKO.SKO_STREET_CHAL,M_BUS_SKO.SKO_WHEEL_TYP_CHAL
  Bus Selector3 : BusSelector  OutputSignals=M_BUS_SKO.SKO_STREET_CHAL
  Display{,1..3} (4 alike) : Display
  Divide{8..14} (7 alike) : Product  Inputs=*/*
  Multiport Switch : MultiPortSwitch  Inputs=7  SaturateOnIntegerOverflow=off  InputSameDT=off
  Multiport Switch2 : MultiPortSwitch  Inputs=7  SaturateOnIntegerOverflow=off  InputSameDT=off
  Multiport Switch3 : MultiPortSwitch  Inputs=4  SaturateOnIntegerOverflow=off  InputSameDT=off
  PS-Simulink Converter{4..10} (7 alike) : nesl_utility/PS-Simulink Converter  PhysicalDomain=network_engine_domain  SubClassName=ps_output  LeftPortType=input  RightPortType=output  PseudoPeriodic=off  Frequencies=[]  VectorFormat=inherit  Unit=inherit  AffineConversion=off
  Scope2 : Scope  NumInputPorts=2
  Simulink-PS Converter5 : nesl_utility/Simulink-PS Converter  PhysicalDomain=network_engine_domain  SubClassName=ps_input  LeftPortType=input  RightPortType=output  PseudoPeriodic=off  Frequencies=[]  NoiseDistribution=none  NoiseParameters=[]  Unit=1  AffineConversion=off  FilteringAndDerivatives=provide  SimscapeFilterOrder=1  InputFilterTimeConstant=0.001  UdotUserProvided=0
  Solver Configuration4 : nesl_utility/Solver Configuration  PhysicalDomain=network_engine_domain  SubClassName=solver  LeftPortType=input  RightPortType=generic  Tones=[]  Harmonics=[]  SimulateNoise=off  Profile=off  UseLocalSampling=off  EnableSwitchedLinearOptims=on  FrequencyDomain=off  UseCCode=off  RelTol=0.001  AbsTol=0.001  MinStep=1e-09  ToWorkspace=off  RevertToSquareIcSolve=off  NumHomotopyIterations=100  PhasorMode=off  PhasorModeNumHarmonics=1  ConsistencySolver=NEWTON_FTOL  CanonicalOrdering=UNORDERED  OptimizeIntermediates=UNOPTIMIZED  IndexReductionMethod=DerivativeReplacement  DoDC=off  ResidualTolerance=1e-09  ConsistencyTolSource=GLOBAL  ConsistencyAbsTol=0.001  ConsistencyRelTol=0.001  ConsistencyTolFactor=0.001  UseLocalSolver=off  LocalSolverChoice=NE_BACKWARD_EULER_ADVANCER  ResolveIndetEquations=on  FunctionEvalNumThread=1  LocalSolverSampleTime=0.001  DoFixedCost=off  MaxNonlinIter=3  MaxModeIter=2  ComputeImpulses=off  ImpulseIterations=2  LinearAlgebra=auto  LinearAlgebraNumThread=0  EquationFormulation=NE_TIME_EF  DelaysMemoryBudget=1024  AutomaticFiltering=on  FilteringTimeConstant=0.001  PartitionStorageMethod=AS_NEEDED  PartitionMemoryBudget=1024  PartitionMethod=ROBUST  MultibodyUseLocalSolver=off  MultibodyLocalSolverChoice=ODE1  MultibodyLocalSolverSampleTime=0.001
  mü  Sportleifen (Pilot Sport) : Constant  Value=1.1
  "mü Eis " : fl_lib/Physical Signals/Lookup Tables/PS Lookup Table (1D)  x=|  f=|  interp_method=simscape.enum.interpolation.smooth  extrap_method=simscape.enum.extrapolation.nearest
      x=|
      | [0
      | 4
      | 8
      | 12
      | 16
      | 20
      | 24
      | 50
      | 80
      | 90
      | 100
      | ]
      f=|
      | [ 0
      | 0.06
      | 0.09
      | 0.1
      | 0.1
      | 0.1
      | 0.1
      | 0.1
      | 0.05
      | 0.02
      | 0.015
      |  ]
  mü Performance Reifen (Corsa) : Constant  Value=1.2
  mü Schnee : fl_lib/Physical Signals/Lookup Tables/PS Lookup Table (1D)  x=|  f=|  interp_method=simscape.enum.interpolation.smooth  extrap_method=simscape.enum.extrapolation.nearest
      x=|
      | [0
      | 4
      | 8
      | 12
      | 16
      | 20
      | 24
      | 50
      | 80
      | 90
      | 100
      | ]
      f=|
      | [ 0
      | 0.08
      | 0.13
      | 0.18
      | 0.2
      | 0.2
      | 0.2
      | 0.2
      | 0.2
      | 0.215
      | 0.27
      | ]
  mü Spezialreifen  (Tropheo) : Constant  Value=1.3
  mü Standardreifen : Constant
  mü max Asphalt nass : Constant  Value=0.81
  mü max Asphalt trocken : Constant  Value=1.18
  mü max Beton nass : Constant  Value=0.84
  mü max Beton trocken : Constant  Value=1.03
  mü max Eis : Constant  Value=0.1
  mü max Schnee : Constant  Value=0.27
  "mü max Schotter " : Constant  Value=0.38
  mü nass Asphalt : fl_lib/Physical Signals/Lookup Tables/PS Lookup Table (1D)  x=|  f=|  interp_method=simscape.enum.interpolation.smooth  extrap_method=simscape.enum.extrapolation.nearest
      x=|
      | [0
      | 4
      | 8
      | 12
      | 16
      | 20
      | 24
      | 50
      | 80
      | 90
      | 100
      | ]
      f=|
      | [  0.000
      | 0.550
      | 0.750
      | 0.800
      | 0.810
      | 0.800
      | 0.780
      | 0.690
      | 0.580
      | 0.540
      | 0.500
      |  ]
  mü nass Beton : fl_lib/Physical Signals/Lookup Tables/PS Lookup Table (1D)  x=|  f=|  interp_method=simscape.enum.interpolation.smooth  extrap_method=simscape.enum.extrapolation.nearest
      x=|
      | [0
      | 4
      | 8
      | 12
      | 16
      | 20
      | 24
      | 50
      | 80
      | 90
      | 100
      | ]
      f=|
      | [ 0
      | 0.6
      | 0.82
      | 0.84
      | 0.83
      | 0.78
      | 0.73
      | 0.6
      | 0.54
      | 0.53
      | 0.52
      | ]
  mü nass Schotter : fl_lib/Physical Signals/Lookup Tables/PS Lookup Table (1D)  x=|  f=|  interp_method=simscape.enum.interpolation.smooth  extrap_method=simscape.enum.extrapolation.nearest
      x=|
      | [0
      | 4
      | 8
      | 12
      | 16
      | 20
      | 24
      | 50
      | 80
      | 90
      | 100
      | ]
      f=|
      | [ 0.000
      | 0.200
      | 0.350
      | 0.380
      | 0.375
      | 0.365
      | 0.360
      | 0.320
      | 0.290
      | 0.280
      | 0.270
      | ]
  mü trocken Asphalt : fl_lib/Physical Signals/Lookup Tables/PS Lookup Table (1D)  x=|  f=|  interp_method=simscape.enum.interpolation.smooth  extrap_method=simscape.enum.extrapolation.nearest
      x=|
      | [0
      | 4
      | 8
      | 12
      | 16
      | 20
      | 24
      | 50
      | 80
      | 90
      | 100
      | ]
      f=|
      | [  0.000
      | 0.930
      | 1.100
      | 1.180
      | 1.170
      | 1.160
      | 1.140
      | 1.010
      | 0.860
      | 0.810
      | 0.750
      | ]
  mü trocken Beton : fl_lib/Physical Signals/Lookup Tables/PS Lookup Table (1D)  x=|  f=|  interp_method=simscape.enum.interpolation.smooth  extrap_method=simscape.enum.extrapolation.nearest
      x=|
      | [0
      | 4
      | 8
      | 12
      | 16
      | 20
      | 24
      | 50
      | 80
      | 90
      | 100
      | ]
      f=|
      | [ 0
      | 0.8
      | 0.97
      | 1.03
      | 0.98
      | 0.92
      | 0.86
      | 0.73
      | 0.72
      | 0.73
      | 0.75
      | ]
  "mü f(s, Fahrbahn)" : Outport
  mü f(Reifen) : Outport  Port=2
  mü eff (s,FB;RF)1 : Outport  Port=3
  wires:
  mü max Beton nass/1 -> Divide11/2
  "mü max Schotter "/1 -> Divide12/2
  Divide8/1 -> Multiport Switch2/2
  Divide10/1 -> Multiport Switch2/4
  Divide11/1 -> Multiport Switch2/5
  s max (%)/1 -> Simulink-PS Converter5/1
  mü Standardreifen/1 -> Multiport Switch3/2
  Divide13/1 -> Multiport Switch2/7
  mü Spezialreifen  (Tropheo)/1 -> Multiport Switch3/4
  PS-Simulink Converter6/1 -> Divide13/1, Multiport Switch/7
  mü max Schnee/1 -> Divide13/2
  mü max Asphalt trocken/1 -> Divide8/2
  X_BUS_CHAL/1 -> Bus Selector1/1, Bus Selector3/1
  PS-Simulink Converter7/1 -> Divide14/1, Multiport Switch/8
  PS-Simulink Converter10/1 -> Divide12/1, Multiport Switch/6
  Bus Selector1/2 -> Display1/1, Multiport Switch3/1  "<SKO_WHEEL_TYP_CHAL>"
  mü Performance Reifen (Corsa)/1 -> Multiport Switch3/3
  PS-Simulink Converter5/1 -> Divide11/1, Multiport Switch/5
  mü max Asphalt nass/1 -> Divide10/2
  PS-Simulink Converter4/1 -> Divide9/1, Multiport Switch/3
  Bus Selector3/1 -> Multiport Switch/1  "<SKO_STREET_CHAL>"
  Bus Selector1/1 -> Display/1, Multiport Switch2/1  "<SKO_STREET_CHAL>"
  Multiport Switch3/1 -> mü f(Reifen)/1, Divide13/3, Divide14/3, Divide12/3, Divide11/3, Divide10/3, Divide9/3, Divide8/3  "mü f(Reifen)"
  Divide9/1 -> Multiport Switch2/3
  Multiport Switch/1 -> "mü f(s, Fahrbahn)"/1  "mü f(s, Fahrbahn)"
  PS-Simulink Converter8/1 -> Divide8/1, Multiport Switch/2
  Multiport Switch2/1 -> Display3/1, Scope2/1, mü eff (s,FB;RF)1/1  "mü eff (s,FB;RF)"
  Divide12/1 -> Multiport Switch2/6
  Divide14/1 -> Display2/1, Scope2/2, Multiport Switch2/8
  mü max Beton trocken/1 -> Divide9/2
  mü  Sportleifen (Pilot Sport)/1 -> Multiport Switch3/5
  PS-Simulink Converter9/1 -> Divide10/1, Multiport Switch/4
  mü max Eis/1 -> Divide14/2
  connections:
  mü Schnee/LConn1 -- "mü Eis "/LConn1 -- mü nass Schotter/LConn1 -- mü nass Beton/LConn1 -- Solver Configuration4/RConn1 -- mü nass Asphalt/LConn1 -- mü trocken Beton/LConn1 -- mü trocken Asphalt/LConn1 -- Simulink-PS Converter5/RConn1
  "mü Eis "/RConn1 -- PS-Simulink Converter7/LConn1
  mü trocken Beton/RConn1 -- PS-Simulink Converter4/LConn1
  mü Schnee/RConn1 -- PS-Simulink Converter6/LConn1
  mü trocken Asphalt/RConn1 -- PS-Simulink Converter8/LConn1
  mü nass Schotter/RConn1 -- PS-Simulink Converter10/LConn1
  mü nass Asphalt/RConn1 -- PS-Simulink Converter9/LConn1
  mü nass Beton/RConn1 -- PS-Simulink Converter5/LConn1
